simulink model "Calculator"  (R2021a)
settings: Solver=FixedStepAuto  StartTime=0.0  StopTime=10.0  RelTol=1e-3
libraries: simulink x2
settings Model: Creator=NoteBook  LastModifiedBy=NoteBook
settings OptimizationCC: DefaultParameterBehavior=Inlined  EnhancedBackFolding=on  PassReuseOutputArgsAs=Individual arguments  ZeroExternalMemoryAtStartup=off  ZeroInternalMemoryAtStartup=off  OptimizeBlockOrder=speed  DifferentSizesBufferReuse=on  OptimizationCustomize=off  EfficientTunableParamExpr=on
settings DebuggingCC: ParameterTunabilityLossMsg=error
settings SFSimCC: MATLABDynamicMemAlloc=off
settings RTWCC: SystemTargetFile=ert.tlc  GenCodeOnly=on  TemplateMakefile=ert_default_tmf  GenerateReport=on  LaunchReport=on
settings CodeAppCC: ForceParamTrailComments=on  IgnoreCustomStorageClasses=off  OperatorAnnotations=on  SimulinkDataObjDesc=on  SFDataObjDesc=on  InsertBlockDesc=on
settings ERTTargetCC: TargetLangStandard=C99 (ISO)  GenerateSampleERTMain=on  InlinedParameterPlacement=NonHierarchical  ERTCustomFileTemplate=example_file_process.tlc

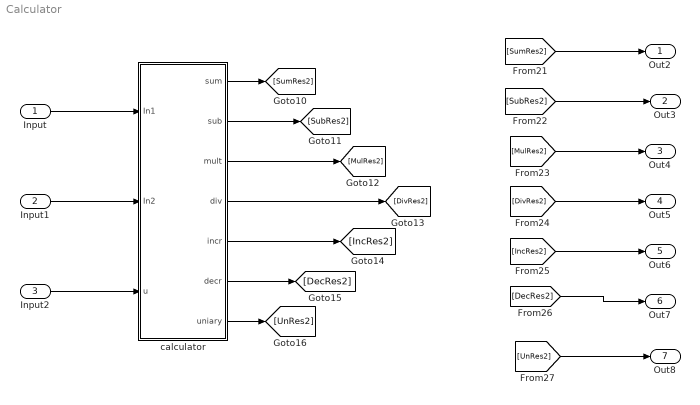
== system Calculator ==
  Input : Inport
  Input1 : Inport  Port=2
  Input2 : Inport  Port=3
  calculator : Subsystem
  Out2 : Outport
  Out3 : Outport  Port=2
  Out4 : Outport  Port=3
  Out5 : Outport  Port=4
  Out6 : Outport  Port=5
  Out7 : Outport  Port=6
  Out8 : Outport  Port=7
  wires:
  calculator/4(div) -> [DivRes2]
  Input2/1 -> calculator/3(u)
  calculator/5(incr) -> [IncRes2]
  calculator/7(uniary) -> [UnRes2]
  [UnRes2] -> Out8/1
  [SubRes2] -> Out3/1
  [DecRes2] -> Out7/1
  [MulRes2] -> Out4/1
  calculator/2(sub) -> [SubRes2]
  [SumRes2] -> Out2/1
  calculator/1(sum) -> [SumRes2]
  Input1/1 -> calculator/2(In2)
  [DivRes2] -> Out5/1
  [IncRes2] -> Out6/1
  calculator/6(decr) -> [DecRes2]
  Input/1 -> calculator/1(In1)
  calculator/3(mult) -> [MulRes2]

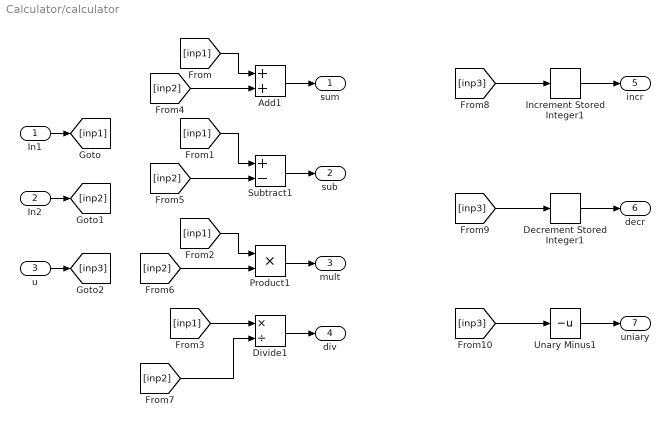
== system Calculator/calculator ==
  In1 : Inport
  In2 : Inport  Port=2
  u : Inport  Port=3
  Add1 : Sum
  Decrement Stored Integer1 : simulink/Additional Math & Discrete/Additional Math: Increment - Decrement/Decrement Stored Integer
      settings: SourceProductBaseCode=SL
  Divide1 : Product  Inputs=*/
  Increment Stored Integer1 : simulink/Additional Math & Discrete/Additional Math: Increment - Decrement/Increment Stored Integer
  Product1 : Product
  Subtract1 : Sum  Inputs=+-
  Unary Minus1 : UnaryMinus
  sum : Outport
  sub : Outport  Port=2
  mult : Outport  Port=3
  div : Outport  Port=4
  incr : Outport  Port=5
  decr : Outport  Port=6
  uniary : Outport  Port=7
  wires:
  Increment Stored Integer1/1 -> incr/1
  Divide1/1 -> div/1
  Subtract1/1 -> sub/1
  Decrement Stored Integer1/1 -> decr/1
  Add1/1 -> sum/1
  Unary Minus1/1 -> uniary/1
  Product1/1 -> mult/1
  u/1 -> [inp3]
  In2/1 -> [inp2]
  In1/1 -> [inp1]
  [inp1] -> Product1/1
  [inp1] -> Add1/1
  [inp1] -> Subtract1/1
  [inp1] -> Divide1/1
  [inp2] -> Add1/2
  [inp2] -> Subtract1/2
  [inp2] -> Product1/2
  [inp2] -> Divide1/2
  [inp3] -> Increment Stored Integer1/1
  [inp3] -> Decrement Stored Integer1/1
  [inp3] -> Unary Minus1/1
